simulink model "RLS"  (R2022b)
settings: Solver=FixedStepAuto  StartTime=0.0  StopTime=t  FixedStep=1  RelTol=1e-3
values from neighbouring files (symbols this model uses):
  Cq = -sum(sum(I_HPPC(I_HPPC<=0)))/3600    [RLS_0730.m]
  f_OCV = polyfit(SOC,V_OCV,index)    [RLS_0730.m]
libraries: matrix_library x1
settings Model: Creator=liull  LastModifiedBy=liull

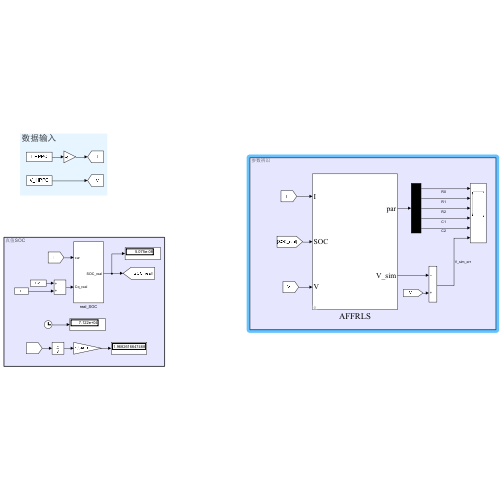
[thumbnail: Simulink's stored preview of the top-level diagram]
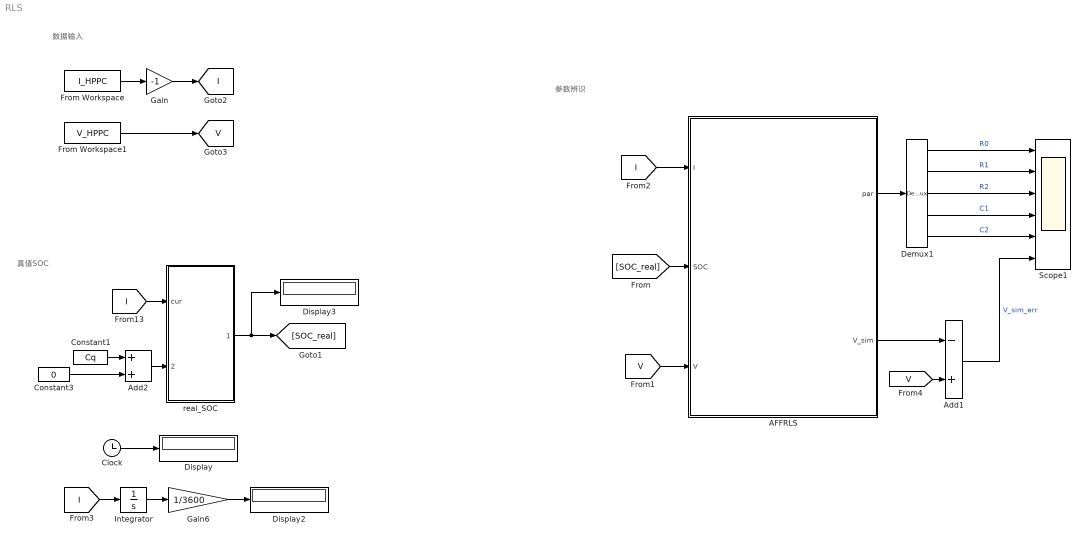
== system RLS ==
  note: 数据输入
  note: 真值SOC
  note: 参数辨识
  AFFRLS : Subsystem  mask{f_OCV=f_OCV, mu_AFFRLS=10000, inter_AFFRLS=4, ff_min_AFFRLS=0.98, P0=100*[1,1,1,1,1]}
      mask prompts: f_OCV "开路电压对SOC的函数"; mu_AFFRLS "ff修正系数mu"; inter_AFFRLS "修正值进位数inter"; ff_min_AFFRLS "ff最小值ff_min"; P0 "初始协方差矩阵P0"
      mask DialogControl DescGroupVar Prompt: AFFRLS
      mask DialogControl ParameterGroupVar Prompt: 参数设置
  Add1 : Sum  Inputs=-+
  Add2 : Sum
  Clock : Clock
  Constant1 : Constant  Value=Cq
  Constant3 : Constant  Value=0
  Demux1 : Demux  Outputs=5
  Display : Display
  Display2 : Display
  Display3 : Display
  From Workspace : FromWorkspace  VariableName=I_HPPC
  From Workspace1 : FromWorkspace  VariableName=V_HPPC
  Gain : Gain  Gain=-1
  Gain6 : Gain  Gain=1/3600
  Integrator : Integrator
  Scope1 : Scope  NumInputPorts=6
  real_SOC : Subsystem
  tag scope: I=global, V=global
  wires:
  From Workspace1/1 -> [V]
  From Workspace/1 -> Gain/1
  Integrator/1 -> Gain6/1
  real_SOC/1(SOC_real) -> Display3/1, [SOC_real]
  [I] -> real_SOC/1(cur)
  [I] -> Integrator/1
  Gain6/1 -> Display2/1
  Clock/1 -> Display/1
  Constant1/1 -> Add2/1
  Add2/1 -> real_SOC/2(Cq_real)
  Constant3/1 -> Add2/2
  Demux1/4 -> Scope1/4  "C1"
  Add1/1 -> Scope1/6  "V_sim_err"
  AFFRLS/1(par) -> Demux1/1
  Demux1/2 -> Scope1/2  "R1"
  Demux1/5 -> Scope1/5  "C2"
  Demux1/1 -> Scope1/1  "R0"
  Demux1/3 -> Scope1/3  "R2"
  [V] -> Add1/2
  AFFRLS/2(V_sim) -> Add1/1
  [V] -> AFFRLS/3(V)
  [SOC_real] -> AFFRLS/2(SOC)
  [I] -> AFFRLS/1(I)
  Gain/1 -> [I]

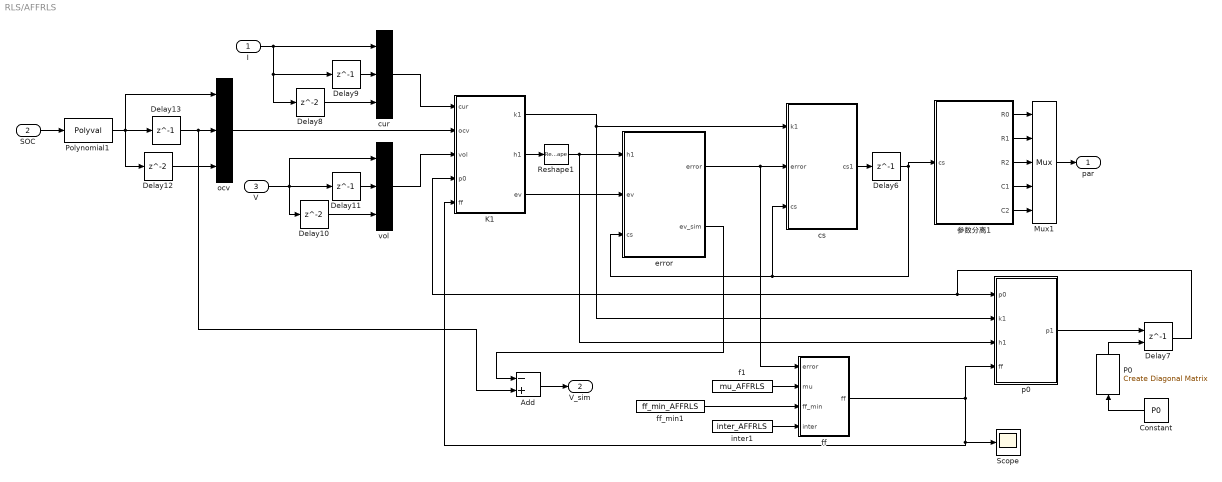
== system RLS/AFFRLS ==
  I : Inport
  SOC : Inport  Port=2
  V : Inport  Port=3
  Add : Sum  Inputs=-+
  Constant : Constant  Value=P0
  Delay10 : Delay  InitialCondition=4.18
  Delay11 : Delay  DelayLength=1  InitialCondition=4.18
  Delay12 : Delay  InitialCondition=4.18
  Delay13 : Delay  DelayLength=1  InitialCondition=4.18
  Delay6 : Delay  DelayLength=1  InitialCondition=[0.1 0.1 0.1 0.1 0.1]'
  Delay7 : Delay  DelayLength=1  InitialConditionSource=Input port  InitialCondition=10^(2)*eye(5,5)
      settings: InputPortMap=u0,p4
  Delay8 : Delay  InitialCondition=0
  Delay9 : Delay  DelayLength=1  InitialCondition=0
  K1 : MATLAB Function  TreatAsAtomicUnit=on
  Mux1 : Mux  Inputs=5
  P0 : matrix_library/Create Diagonal Matrix
  Polynomial1 : Polyval  Coefs=f_OCV
  Reshape1 : Reshape  OutputDimensionality=Customize  OutputDimensions=[5,1]
  Scope : Scope
  cs : MATLAB Function  TreatAsAtomicUnit=on
  cur : Mux  Inputs=3
  error : MATLAB Function  TreatAsAtomicUnit=on
  f1 : Constant  Value=mu_AFFRLS
  ff : Subsystem
  ff_min1 : Constant  Value=ff_min_AFFRLS
  inter1 : Constant  Value=inter_AFFRLS
  ocv : Mux  Inputs=3
  p0 : MATLAB Function  TreatAsAtomicUnit=on
  vol : Mux  Inputs=3
  参数分离1 : MATLAB Function  TreatAsAtomicUnit=on
  par : Outport
  V_sim : Outport  Port=2
  wires:
  p0/1(p1) -> Delay7/1
  Delay6/1 -> 参数分离1/1(cs), error/3(cs), cs/3(cs)
  cur/1 -> K1/1(cur)
  Delay7/1 -> K1/4(p0), p0/1(p0)
  K1/3(ev) -> error/2(ev)
  cs/1(cs1) -> Delay6/1
  V/1 -> Delay10/1, Delay11/1, vol/1
  K1/1(k1) -> cs/1(k1), p0/2(k1)
  ff_min1/1 -> ff/3(ff_min)
  Delay10/1 -> vol/3
  Delay9/1 -> cur/2
  SOC/1 -> Polynomial1/1
  Delay12/1 -> ocv/3
  K1/2(h1) -> Reshape1/1
  f1/1 -> ff/2(mu)
  Delay13/1 -> Add/2, ocv/2
  Delay11/1 -> vol/2
  Delay8/1 -> cur/3
  Polynomial1/1 -> Delay12/1, Delay13/1, ocv/1
  ocv/1 -> K1/2(ocv)
  inter1/1 -> ff/4(inter)
  vol/1 -> K1/3(vol)
  ff/1(ff) -> p0/4(ff), K1/5(ff), Scope/1
  Reshape1/1 -> error/1(h1), p0/3(h1)
  I/1 -> Delay9/1, Delay8/1, cur/1
  参数分离1/1(R0) -> Mux1/1
  参数分离1/2(R1) -> Mux1/2
  参数分离1/3(R2) -> Mux1/3
  参数分离1/4(C1) -> Mux1/4
  参数分离1/5(C2) -> Mux1/5
  Mux1/1 -> par/1
  P0/1 -> Delay7/2
  Constant/1 -> P0/1
  error/1(error) -> ff/1(error), cs/2(error)
  error/2(ev_sim) -> Add/1
  Add/1 -> V_sim/1

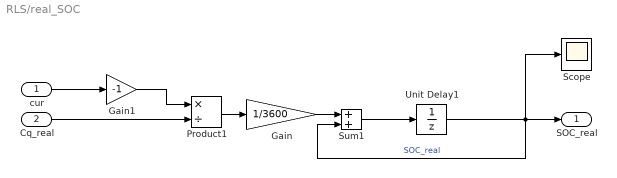
== system RLS/real_SOC ==
  cur : Inport
  Cq_real : Inport  Port=2
  Gain : Gain  Gain=1/3600
  Gain1 : Gain  Gain=-1
  Product1 : Product  Inputs=*/
  Scope : Scope
  Sum1 : Sum
  Unit Delay1 : UnitDelay  InitialCondition=1  SampleTime=-1  HasFrameUpgradeWarning=on
  SOC_real : Outport
  wires:
  cur/1 -> Gain1/1
  Product1/1 -> Gain/1
  Unit Delay1/1 -> Scope/1, Sum1/2, SOC_real/1  "SOC_real"
  Sum1/1 -> Unit Delay1/1
  Cq_real/1 -> Product1/2
  Gain/1 -> Sum1/1
  Gain1/1 -> Product1/1

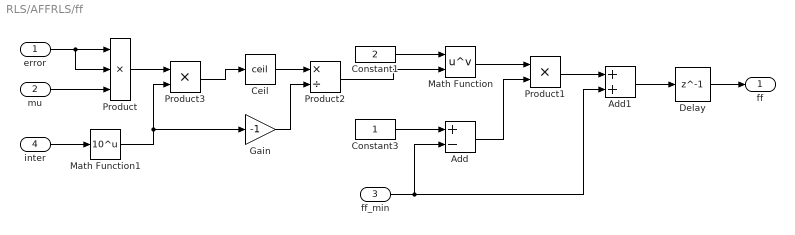
== system RLS/AFFRLS/ff ==
  error : Inport
  mu : Inport  Port=2
  ff_min : Inport  Port=3
  inter : Inport  Port=4
  Add : Sum  Inputs=+-
  Add1 : Sum
  Ceil : Rounding  Operator=ceil
  Constant1 : Constant  Value=2
  Constant3 : Constant
  Delay : Delay  DelayLength=1  InitialCondition=1
  Gain : Gain  Gain=-1
  Math Function : Math  Operator=pow  SignedPower=on
  Math Function1 : Math  Operator=10^u  SignedPower=on
  Product : Product  Inputs=3
  Product1 : Product
  Product2 : Product  Inputs=*/
  Product3 : Product
  ff : Outport
  wires:
  Product2/1 -> Math Function/2
  Product/1 -> Product3/1
  ff_min/1 -> Add1/2, Add/2
  Math Function/1 -> Product1/1
  Ceil/1 -> Product2/1
  mu/1 -> Product/3
  Constant3/1 -> Add/1
  Product1/1 -> Add1/1
  Add/1 -> Product1/2
  Constant1/1 -> Math Function/1
  Product3/1 -> Ceil/1
  error/1 -> Product/1, Product/2
  Add1/1 -> Delay/1
  Delay/1 -> ff/1
  Gain/1 -> Product2/2
  Math Function1/1 -> Product3/2, Gain/1
  inter/1 -> Math Function1/1

== matlab function RLS/AFFRLS/K1 ==
  data: cur input; ocv input; k1 output; vol input; p0 input; ff input; h1 output; ev output
function [k1,h1,ev] = RLS_identify(cur,ocv,vol,p0,ff)
ev=ocv-vol;
h1=[ev(2),ev(3),cur(1),cur(2),cur(3)]';
q=h1'*p0*h1+ff;
k1=p0*h1/q;              
end

== matlab function RLS/AFFRLS/cs ==
  data: k1 input; error input; cs1 output; cs input
function cs1=RLS_identify(k1,error,cs)
cs1=cs+k1*error;
end

== matlab function RLS/AFFRLS/error ==
  data: h1 input; ev input; error output; cs input; ev_sim output
function [error,ev_sim]=RLS_identify(h1,ev,cs)
ev_sim=h1'*cs;
error=ev(1)-ev_sim;        %求电压实验值和理论值误差
end

== matlab function RLS/AFFRLS/p0 ==
  data: p0 input; k1 input; p1 output; h1 input; ff input
function p1=RLS_identify(p0,k1,h1,ff)
p1=(p0-k1*h1'*p0)/ff;
end

== matlab function RLS/AFFRLS/参数分离1 ==
  data: R0 output; R1 output; cs input; R2 output; C1 output; C2 output
function [R0,R1,R2,C1,C2]= get_paras(cs)
%% 分离参数
T = 1;
a1=cs(1); a2=cs(2); a3=cs(3); a4=cs(4); a5=cs(5);

b0=(a3-a4+a5)./(1+a1-a2);
b1=T*T*(1+a1-a2)./(4*(1-a1-a2));
b2=T*(1+a2)./(1-a1-a2);
b3=(a3+a4+a5)./(1-a1-a2);
b4=T*(a3-a5)./(1-a1-a2);

dd=b2.*b2-4*b1;
tsp=[(b2+sqrt(dd))/2;(b2-sqrt(dd))/2];

R0=(b0);
t2=tsp(1,:);
t1=tsp(2,:);
R2=(b4-R0.*t1-b3.*t2)./(t1-t2);
R1=b3-R0-R2;
C2=t2./R2;
C1=t1./R1;
end
